simulink model "PI_Laengsregler"  (R2019b)
settings: Solver=VariableStepAuto  StartTime=0.0  StopTime=500  MaxStep=0.01  RelTol=1e-3

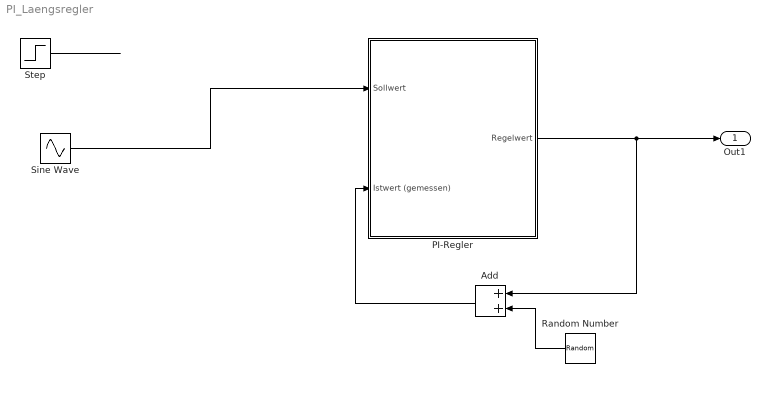
== system PI_Laengsregler ==
  Add : Sum
  PI-Regler : Subsystem
  Random Number : RandomNumber  Variance=0.1  SampleTime=0.1
  Sine Wave : Sin  Frequency=10  SampleTime=0
  Step : Step  SampleTime=0
  Out1 : Outport  VectorParamsAs1DForOutWhenUnconnected=off
  wires:
  Step/1 -> ?
  PI-Regler/1(Regelwert) -> Add/1, Out1/1
  Random Number/1 -> Add/2
  Add/1 -> PI-Regler/2(Istwert (gemessen))
  Sine Wave/1 -> PI-Regler/1(Sollwert)

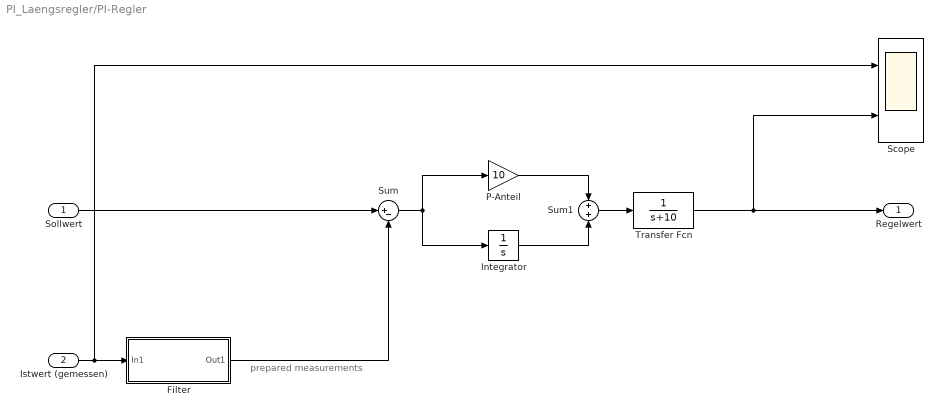
== system PI_Laengsregler/PI-Regler ==
  note: prepared measurements
  Sollwert : Inport
  Istwert (gemessen) : Inport  Port=2
  "Filter " : Subsystem
  Integrator : Integrator
  "P-Anteil " : Gain  Gain=10
  Scope : Scope  NumInputPorts=2
  Sum : Sum  Inputs=|+-
  Sum1 : Sum  Inputs=+|+
  Transfer Fcn : TransferFcn  Denominator=[1 10]
  Regelwert : Outport  VectorParamsAs1DForOutWhenUnconnected=off
  wires:
  Sum/1 -> Integrator/1, "P-Anteil "/1
  Integrator/1 -> Sum1/2
  "P-Anteil "/1 -> Sum1/1
  Sum1/1 -> Transfer Fcn/1
  Transfer Fcn/1 -> Scope/2, Regelwert/1
  Istwert (gemessen)/1 -> Scope/1, "Filter "/1(In1)
  "Filter "/1(Out1) -> Sum/2
  Sollwert/1 -> Sum/1

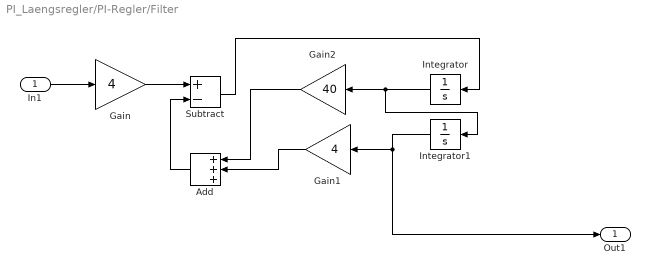
== system PI_Laengsregler/PI-Regler/Filter  ==
  In1 : Inport
  Add : Sum  Inputs=3
  Gain : Gain  Gain=4
  Gain1 : Gain  Gain=4
  Gain2 : Gain  Gain=40
  Integrator : Integrator
  Integrator1 : Integrator
  Subtract : Sum  Inputs=+-
  Out1 : Outport  VectorParamsAs1DForOutWhenUnconnected=off
  wires:
  In1/1 -> Gain/1
  Gain/1 -> Subtract/1
  Add/1 -> Subtract/2
  Gain1/1 -> Add/2
  Gain2/1 -> Add/1
  Integrator/1 -> Integrator1/1, Gain2/1
  Subtract/1 -> Integrator/1
  Integrator1/1 -> Out1/1, Gain1/1
